simulink model "Simulation"  (R2016a)
settings: Solver=FixedStepAuto  StartTime=0.0  StopTime=20  FixedStep=0.01  RelTol=1e-3
undefined symbols (not defined in the file or in its folder): beta, g0, g1, g2, g3, gamma, kappa, landa, nu
(part 2 of 30)

== matlab function Simulation/Ueq ==
  data: e input; edot input; xddd input; despar input; landa input; S input; y1 output; theta input; thetadot input; y2 output; y3 output; y4 output; y5 output; y6 output
function [y1,y2,y3,y4,y5,y6] = fcn(e,edot,xddd,despar,landa,S,theta,thetadot)

y=zeros(6,1)
p1=despar(1)*((abs(e(1)))^despar(5))*sign(e(1))+despar(2)*e(1)+despar(3)*despar(6)*(abs(e(1)))^(despar(6)-1)*edot(1);
p2=despar(1)*((abs(e(2)))^despar(5))*sign(e(2))+despar(2)*e(2)+despar(3)*despar(6)*(abs(e(2)))^(despar(6)-1)*edot(2);
p3=despar(1)*((abs(e(3)))^despar(5))*sign(e(3))+despar(2)*e(3)+despar(3)*despar(6)*(abs(e(3)))^(despar(6)-1)*edot(3);
p4=despar(1)*((abs(e(4)))^despar(5))*sign(e(4))+despar(2)*e(4)+despar(3)*despar(6)*(abs(e(4)))^(despar(6)-1)*edot(4);
p5=despar(1)*((abs(e(5)))^despar(5))*sign(e(5))+despar(2)*e(5)+despar(3)*despar(6)*(abs(e(5)))^(despar(6)-1)*edot(5);
p6=despar(1)*((abs(e(6)))^despar(5))*sign(e(6))+despar(2)*e(6)+despar(3)*despar(6)*(abs(e(6)))^(despar(6)-1)*edot(6);

part=[p1 p2 p3 p4 p5 p6]';

theta1=theta(1)
theta2=theta(2)
theta3=theta(3)
theta4=theta(4)
theta5=theta(5)
theta6=theta(6)

thetadot1=thetadot(1)
thetadot2=thetadot(2)
thetadot3=thetadot(3)
thetadot4=thetadot(4)
thetadot5=thetadot(5)
thetadot6=thetadot(6)

MM=[ 0.1*cos(theta2 + theta3)^2 + (0.1*cos(theta2)*cos(theta3)*cos(theta6)*sin(theta4) - 0.1*cos(theta6)*sin(theta2)*sin(theta3)*sin(theta4) + 0.1*cos(theta2)*sin(theta3)*sin(theta5)*sin(theta6) + 0.1*cos(theta3)*sin(theta2)*sin(theta5)*sin(theta6) - 0.1*cos(theta2)*cos(theta3)*cos(theta4)*cos(theta5)*sin(theta6) + 0.1*cos(theta4)*cos(theta5)*sin(theta2)*sin(theta3)*sin(theta6))*(cos(theta2)*cos(theta3)*cos(theta6)*sin(theta4) - 1.0*cos(theta6)*sin(theta2)*sin(theta3)*sin(theta4) + cos(theta2)*sin(theta3)*sin(theta5)*sin(theta6) + cos(theta3)*sin(theta2)*sin(theta5)*sin(theta6) - 1.0*cos(theta2)*cos(theta3)*cos(theta4)*cos(theta5)*sin(theta6) + cos(theta4)*cos(theta5)*sin(theta2)*sin(theta3)*sin(theta6)) + 0.2*sin(theta2 + theta3)^2 + (0.2*cos(theta2)*sin(theta4)*sin(theta5) + 0.4*sin(theta2)*sin(theta3)*sin(theta4) - 0.4*cos(theta2)*cos(theta3)*sin(theta4) + 0.4*cos(theta2)*cos(theta3)*cos(theta6)*sin(theta4) + 0.4*cos(theta2)*cos(theta3)*sin(theta4)*sin(theta5) - 0.4*cos(theta6)*sin(theta2)*sin(theta3)*sin(theta4) + 0.4*cos(theta2)*sin(theta3)*sin(theta5)*sin(theta6) + 0.4*cos(theta3)*sin(theta2)*sin(theta5)*sin(theta6) - 0.4*sin(theta2)*sin(theta3)*sin(theta4)*sin(theta5) - 0.4*cos(theta2)*cos(theta3)*cos(theta4)*cos(theta5)*sin(theta6) + 0.4*cos(theta4)*cos(theta5)*sin(theta2)*sin(theta3)*sin(theta6))^2 + 0.14*cos(theta2)^2 + 0.1*sin(theta2)^2 + (cos(theta2)*sin(theta3)*sin(theta5) + cos(theta3)*sin(theta2)*sin(theta5) - 1.0*cos(theta2)*cos(theta3)*cos(theta4)*cos(theta5) + cos(theta4)*cos(theta5)*sin(theta2)*sin(theta3))*(0.1*cos(theta2)*sin(theta3)*sin(theta5) + 0.1*cos(theta3)*sin(theta2)*sin(theta5) - 0.1*cos(theta2)*cos(theta3)*cos(theta4)*cos(theta5) + 0.1*cos(theta4)*cos(theta5)*sin(theta2)*sin(theta3)) + 2.0*(cos(theta2)*cos(theta5)*sin(theta3) + cos(theta3)*cos(theta5)*sin(theta2) + cos(theta2)*cos(theta3)*cos(theta4)*sin(theta5) - 1.0*cos(theta4)*sin(theta2)*sin(theta3)*sin(theta5))*(0.1*cos(theta2)*cos(theta5)*sin(theta3) + 0.1*cos(theta3)*cos(theta5)*sin(theta2) + 0.1*cos(theta2)*cos(theta3)*cos(theta4)*sin(theta5) - 0.1*cos(theta4)*sin(theta2)*sin(theta3)*sin(theta5)) + 0.04*cos(theta4)^2*(2.0*cos(theta2 + theta3) + cos(theta2))^2 + 0.1*cos(theta2 + theta3)^2*cos(theta4)^2 + 0.2*cos(theta2 + theta3)^2*sin(theta4)^2 + (0.1*cos(theta2)*cos(theta6)*sin(theta3)*sin(theta5) - 0.1*cos(theta2)*cos(theta3)*sin(theta4)*sin(theta6) + 0.1*cos(theta3)*cos(theta6)*sin(theta2)*sin(theta5) + 0.1*sin(theta2)*sin(theta3)*sin(theta4)*sin(theta6) - 0.1*cos(theta2)*cos(theta3)*cos(theta4)*cos(theta5)*cos(theta6) + 0.1*cos(theta4)*cos(theta5)*cos(theta6)*sin(theta2)*sin(theta3))*(cos(theta2)*cos(theta6)*sin(theta3)*sin(theta5) - 1.0*cos(theta2)*cos(theta3)*sin(theta4)*sin(theta6) + cos(theta3)*cos(theta6)*sin(theta2)*sin(theta5) + sin(theta2)*sin(theta3)*sin(theta4)*sin(theta6) - 1.0*cos(theta2)*cos(theta3)*cos(theta4)*cos(theta5)*cos(theta6) + cos(theta4)*cos(theta5)*cos(theta6)*sin(theta2)*sin(theta3)) + 0.04*cos(theta4)^2*(cos(theta2 + theta3) + cos(theta2))^2 + 0.04*sin(theta4)^2*(cos(theta2 + theta3) + cos(theta2))^2 + (0.2*cos(theta2)*cos(theta5)*cos(theta6)*sin(theta4) - 0.4*cos(theta2)*cos(theta3)*cos(theta4)*sin(theta6) - 0.2*cos(theta2)*cos(theta4)*sin(theta6) + 0.4*cos(theta2)*cos(theta5)*sin(theta3)*sin(theta6) + 0.4*cos(theta3)*cos(theta5)*sin(theta2)*sin(theta6) + 0.4*cos(theta4)*sin(theta2)*sin(theta3)*sin(theta6) + 0.4*cos(theta2)*cos(theta3)*cos(theta5)*cos(theta6)*sin(theta4) + 0.4*cos(theta2)*cos(theta3)*cos(theta4)*sin(theta5)*sin(theta6) - 0.4*cos(theta5)*cos(theta6)*sin(theta2)*sin(theta3)*sin(theta4) - 0.4*cos(theta4)*sin(theta2)*sin(theta3)*sin(theta5)*sin(theta6))^2 + (0.2*cos(theta2)*cos(theta4)*cos(theta6) + 0.4*cos(theta2)*cos(theta5)*sin(theta3) + 0.4*cos(theta3)*cos(theta5)*sin(theta2) + 0.4*cos(theta2)*cos(theta3)*cos(theta4)*cos(theta6) + 0.4*cos(theta2)*cos(theta3)*cos(theta4)*sin(theta5) - 0.4*cos(theta2)*cos(theta5)*cos(theta6)*sin(theta3) - 0.4*cos(theta3)*cos(theta5)*cos(theta6)*sin(theta2) - 0.4*cos(theta4)*cos(theta6)*sin(theta2)*sin(theta3) + 0.2*cos(theta2)*cos(theta5)*sin(theta4)*sin(theta6) - 0.4*cos(theta4)*sin(theta2)*sin(theta3)*sin(theta5) - 0.4*cos(theta2)*cos(theta3)*cos(theta4)*cos(theta6)*sin(theta5) + 0.4*cos(theta2)*cos(theta3)*cos(theta5)*sin(theta4)*sin(theta6) + 0.4*cos(theta4)*cos(theta6)*sin(theta2)*sin(theta3)*sin(theta5) - 0.4*cos(theta5)*sin(theta2)*sin(theta3)*sin(theta4)*sin(theta6))^2 + 0.04*cos(theta5)^2*sin(theta4)^2*(2.0*cos(theta2 + theta3) + cos(theta2))^2 + 0.04*sin(theta4)^2*sin(theta5)^2*(2.0*cos(theta2 + theta3) + cos(theta2))^2 + 0.1, 0.16*cos(theta2)*cos(theta3)*cos(theta4)*sin(theta4) - 0.08*cos(theta4)*sin(theta2)*sin(theta6) - 0.08*cos(theta5)*sin(theta2)*sin(theta4) + 0.16*cos(theta2)*cos(theta3)*cos(theta5)*sin(theta6) - 0.16*cos(theta2)*cos(theta5)*sin(theta3)*sin(theta4) - 0.16*cos(theta3)*cos(theta5)*sin(theta2)*sin(theta4) - 0.16*cos(theta2)*cos(theta4)*sin(theta3)*sin(theta6) - 0.16*cos(theta3)*cos(theta4)*sin(theta2)*sin(theta6) + 0.08*cos(theta5)*cos(theta6)*sin(theta2)*sin(theta4) - 0.16*cos(theta4)*sin(theta2)*sin(theta3)*sin(theta4) - 0.16*cos(theta5)*sin(theta2)*sin(theta3)*sin(theta6) - 0.16*cos(theta2)*cos(theta3)*cos(theta4)*cos(theta5)^2*sin(theta4) - 0.16*cos(theta2)*cos(theta3)*cos(theta4)*cos(theta6)^2*sin(theta4) - 0.32*cos(theta2)*cos(theta3)*cos(theta4)^2*cos(theta5)*sin(theta6) + 0.16*cos(theta4)*cos(theta5)^2*sin(theta2)*sin(theta3)*sin(theta4) + 0.16*cos(theta4)*cos(theta6)^2*sin(theta2)*sin(theta3)*sin(theta4) + 0.32*cos(theta4)^2*cos(theta5)*sin(theta2)*sin(theta3)*sin(theta6) - 0.16*cos(theta2)*cos(theta3)*cos(theta5)*cos(theta6)*sin(theta6) + 0.16*cos(theta2)*cos(theta5)*cos(theta6)*sin(theta3)*sin(theta4) + 0.16*cos(theta3)*cos(theta5)*cos(theta6)*sin(theta2)*sin(theta4) + 0.16*cos(theta2)*cos(theta5)*sin(theta3)*sin(theta4)*sin(theta5) + 0.16*cos(theta3)*cos(theta5)*sin(theta2)*sin(theta4)*sin(theta5) + 0.16*cos(theta2)*cos(theta4)*sin(theta3)*sin(theta5)*sin(theta6) + 0.16*cos(theta3)*cos(theta4)*sin(theta2)*sin(theta5)*sin(theta6) + 0.16*cos(theta5)*cos(theta6)*sin(theta2)*sin(theta3)*sin(theta6) - 0.16*cos(theta2)*cos(theta3)*cos(theta4)*cos(theta5)^2*cos(theta6)^2*sin(theta4) + 0.16*cos(theta4)*cos(theta5)^2*cos(theta6)^2*sin(theta2)*sin(theta3)*sin(theta4) - 0.32*cos(theta2)*cos(theta5)*cos(theta6)*sin(theta3)*sin(theta4)*sin(theta5) - 0.32*cos(theta3)*cos(theta5)*cos(theta6)*sin(theta2)*sin(theta4)*sin(theta5) - 0.16*cos(theta2)*cos(theta4)*cos(theta6)*sin(theta3)*sin(theta5)*sin(theta6) - 0.16*cos(theta3)*cos(theta4)*cos(theta6)*sin(theta2)*sin(theta5)*sin(theta6) + 0.32*cos(theta2)*cos(theta3)*cos(theta4)*cos(theta5)^2*cos(theta6)*sin(theta4) + 0.32*cos(theta2)*cos(theta3)*cos(theta4)^2*cos(theta5)*cos(theta6)*sin(theta6) - 0.32*cos(theta4)*cos(theta5)^2*cos(theta6)*sin(theta2)*sin(theta3)*sin(theta4) + 0.16*cos(theta2)*cos(theta5)*cos(theta6)^2*sin(theta3)*sin(theta4)*sin(theta5) + 0.16*cos(theta3)*cos(theta5)*cos(theta6)^2*sin(theta2)*sin(theta4)*sin(theta5) - 0.32*cos(theta4)^2*cos(theta5)*cos(theta6)*sin(theta2)*sin(theta3)*sin(theta6), 0.16*cos(theta2)*cos(theta3)*cos(theta4)*sin(theta4) + 0.16*cos(theta2)*cos(theta3)*cos(theta5)*sin(theta6) - 0.16*cos(theta2)*cos(theta5)*sin(theta3)*sin(theta4) - 0.16*cos(theta3)*cos(theta5)*sin(theta2)*sin(theta4) - 0.16*cos(theta2)*cos(theta4)*sin(theta3)*sin(theta6) - 0.16*cos(theta3)*cos(theta4)*sin(theta2)*sin(theta6) - 0.16*cos(theta4)*sin(theta2)*sin(theta3)*sin(theta4) - 0.16*cos(theta5)*sin(theta2)*sin(theta3)*sin(theta6) - 0.16*cos(theta2)*cos(theta3)*cos(theta4)*cos(theta5)^2*sin(theta4) - 0.16*cos(theta2)*cos(theta3)*cos(theta4)*cos(theta6)^2*sin(theta4) - 0.32*cos(theta2)*cos(theta3)*cos(theta4)^2*cos(theta5)*sin(theta6) + 0.16*cos(theta4)*cos(theta5)^2*sin(theta2)*sin(theta3)*sin(theta4) + 0.16*cos(theta4)*cos(theta6)^2*sin(theta2)*sin(theta3)*sin(theta4) + 0.32*cos(theta4)^2*cos(theta5)*sin(theta2)*sin(theta3)*sin(theta6) - 0.16*cos(theta2)*cos(theta3)*cos(theta5)*cos(theta6)*sin(theta6) + 0.16*cos(theta2)*cos(theta5)*cos(theta6)*sin(theta3)*sin(theta4) + 0.16*cos(theta3)*cos(theta5)*cos(theta6)*sin(theta2)*sin(theta4) + 0.16*cos(theta2)*cos(theta5)*sin(theta3)*sin(theta4)*sin(theta5) + 0.16*cos(theta3)*cos(theta5)*sin(theta2)*sin(theta4)*sin(theta5) + 0.16*cos(theta2)*cos(theta4)*sin(theta3)*sin(theta5)*sin(theta6) + 0.16*cos(theta3)*cos(theta4)*sin(theta2)*sin(theta5)*sin(theta6) + 0.16*cos(theta5)*cos(theta6)*sin(theta2)*sin(theta3)*sin(theta6) - 0.16*cos(theta2)*cos(theta3)*cos(theta4)*cos(theta5)^2*cos(theta6)^2*sin(theta4) + 0.16*cos(theta4)*cos(theta5)^2*cos(theta6)^2*sin(theta2)*sin(theta3)*sin(theta4) - 0.32*cos(theta2)*cos(theta5)*cos(theta6)*sin(theta3)*sin(theta4)*sin(theta5) - 0.32*cos(theta3)*cos(theta5)*cos(theta6)*sin(theta2)*sin(theta4)*sin(theta5) - 0.16*cos(theta2)*cos(theta4)*cos(theta6)*sin(theta3)*sin(theta5)*sin(theta6) - 0.16*cos(theta3)*cos(theta4)*cos(theta6)*sin(theta2)*sin(theta5)*sin(theta6) + 0.32*cos(theta2)*cos(theta3)*cos(theta4)*cos(theta5)^2*cos(theta6)*sin(theta4) + 0.32*cos(theta2)*cos(theta3)*cos(theta4)^2*cos(theta5)*cos(theta6)*sin(theta6) - 0.32*cos(theta4)*cos(theta5)^2*cos(theta6)*sin(theta2)*sin(theta3)*sin(theta4) + 0.16*cos(theta2)*cos(theta5)*cos(theta6)^2*sin(theta3)*sin(theta4)*sin(theta5) + 0.16*cos(theta3)*cos(theta5)*cos(theta6)^2*sin(theta2)*sin(theta4)*sin(theta5) - 0.32*cos(theta4)^2*cos(theta5)*cos(theta6)*sin(theta2)*sin(theta3)*sin(theta6), 0.46*cos(theta2)*sin(theta3) + 0.46*cos(theta3)*sin(theta2) + 0.08*cos(theta2)*sin(theta4)*sin(theta6) + 0.16*cos(theta2)*cos(theta5)^2*sin(theta3) + 0.16*cos(theta3)*cos(theta5)^2*sin(theta2) - 0.16*cos(theta2)*cos(theta6)^2*sin(theta3) - 0.16*cos(theta3)*cos(theta6)^2*sin(theta2) - 0.08*cos(theta2)*cos(theta4)*cos(theta5) - 0.32*cos(theta2)*cos(theta5)^2*cos(theta6)*sin(theta3) - 0.32*cos(theta3)*cos(theta5)^2*cos(theta6)*sin(theta2) + 0.16*cos(theta2)*cos(theta5)^2*cos(theta6)^2*sin(theta3) + 0.16*cos(theta3)*cos(theta5)^2*cos(theta6)^2*sin(theta2) - 0.16*cos(theta2)*cos(theta3)*cos(theta4)*cos(theta5) + 0.08*cos(theta2)*cos(theta4)*cos(theta5)*cos(theta6) + 0.16*cos(theta4)*cos(theta5)*sin(theta2)*sin(theta3) + 0.16*cos(theta2)*cos(theta3)*sin(theta4)*sin(theta6) - 0.16*sin(theta2)*sin(theta3)*sin(theta4)*sin(theta6) + 0.16*cos(theta2)*cos(theta3)*cos(theta4)*cos(theta5)*cos(theta6) + 0.16*cos(theta2)*cos(theta3)*cos(theta4)*cos(theta5)*sin(theta5) - 0.16*cos(theta4)*cos(theta5)*cos(theta6)*sin(theta2)*sin(theta3) - 0.16*cos(theta4)*cos(theta5)*sin(theta2)*sin(theta3)*sin(theta5) - 0.16*cos(theta2)*cos(theta3)*sin(theta4)*sin(theta5)*sin(theta6) + 0.16*sin(theta2)*sin(theta3)*sin(theta4)*sin(theta5)*sin(theta6) - 0.32*cos(theta2)*cos(theta3)*cos(theta4)*cos(theta5)*cos(theta6)*sin(theta5) + 0.32*cos(theta4)*cos(theta5)*cos(theta6)*sin(theta2)*sin(theta3)*sin(theta5) + 0.16*cos(theta2)*cos(theta3)*cos(theta6)*sin(theta4)*sin(theta5)*sin(theta6) - 0.16*cos(theta6)*sin(theta2)*sin(theta3)*sin(theta4)*sin(theta5)*sin(theta6) + 0.16*cos(theta2)*cos(theta3)*cos(theta4)*cos(theta5)*cos(theta6)^2*sin(theta5) - 0.16*cos(theta4)*cos(theta5)*cos(theta6)^2*sin(theta2)*sin(theta3)*sin(theta5), 0.08*cos(theta2)*sin(theta4)*sin(theta5) + 0.36*sin(theta2)*sin(theta3)*sin(theta4) - 0.36*cos(theta2)*cos(theta3)*sin(theta4) - 0.16*cos(theta2)*cos(theta3)*cos(theta6)^2*sin(theta4) + 0.16*cos(theta6)^2*sin(theta2)*sin(theta3)*sin(theta4) + 0.32*cos(theta2)*cos(theta3)*cos(theta6)*sin(theta4) + 0.16*cos(theta2)*cos(theta3)*sin(theta4)*sin(theta5) - 0.08*cos(theta2)*cos(theta6)*sin(theta4)*sin(theta5) - 0.32*cos(theta6)*sin(theta2)*sin(theta3)*sin(theta4) + 0.16*cos(theta2)*sin(theta3)*sin(theta5)*sin(theta6) + 0.16*cos(theta3)*sin(theta2)*sin(theta5)*sin(theta6) - 0.16*sin(theta2)*sin(theta3)*sin(theta4)*sin(theta5) - 0.16*cos(theta2)*cos(theta3)*cos(theta4)*cos(theta5)*sin(theta6) - 0.16*cos(theta2)*cos(theta3)*cos(theta6)*sin(theta4)*sin(theta5) + 0.16*cos(theta4)*cos(theta5)*sin(theta2)*sin(theta3)*sin(theta6) - 0.16*cos(theta2)*cos(theta6)*sin(theta3)*sin(theta5)*sin(theta6) - 0.16*cos(theta3)*cos(theta6)*sin(theta2)*sin(theta5)*sin(theta6) + 0.16*cos(theta6)*sin(theta2)*sin(theta3)*sin(theta4)*sin(theta5) + 0.16*cos(theta2)*cos(theta3)*cos(theta4)*cos(theta5)*cos(theta6)*sin(theta6) - 0.16*cos(theta4)*cos(theta5)*cos(theta6)*sin(theta2)*sin(theta3)*sin(theta6), 0.08*cos(theta2)*cos(theta4)*cos(theta6) + 0.26*cos(theta2)*cos(theta5)*sin(theta3) + 0.26*cos(theta3)*cos(theta5)*sin(theta2) + 0.16*cos(theta2)*cos(theta3)*cos(theta4)*cos(theta6) + 0.26*cos(theta2)*cos(theta3)*cos(theta4)*sin(theta5) - 0.16*cos(theta2)*cos(theta5)*cos(theta6)*sin(theta3) - 0.16*cos(theta3)*cos(theta5)*cos(theta6)*sin(theta2) - 0.16*cos(theta4)*cos(theta6)*sin(theta2)*sin(theta3) + 0.08*cos(theta2)*cos(theta5)*sin(theta4)*sin(theta6) - 0.26*cos(theta4)*sin(theta2)*sin(theta3)*sin(theta5) - 0.16*cos(theta2)*cos(theta3)*cos(theta4)*cos(theta6)*sin(theta5) + 0.16*cos(theta2)*cos(theta3)*cos(theta5)*sin(theta4)*sin(theta6) + 0.16*cos(theta4)*cos(theta6)*sin(theta2)*sin(theta3)*sin(theta5) - 0.16*cos(theta5)*sin(theta2)*sin(theta3)*sin(theta4)*sin(theta6);
                                                                                                                                                                                                                                                                                                                                                                                                                                                                                                                                                                                                                                                                                                                                                                                                                                                                                                                                                                                                                                                                                                                                                                                                                                                                                                                                                                                                                                                                                                                                                                                                                                                                                                                                                                                                                                                                                                                                                                                                                                                                                                                                                                       0.16*cos(theta2)*cos(theta3)*cos(theta4)*sin(theta4) - 0.08*cos(theta4)*sin(theta2)*sin(theta6) - 0.08*cos(theta5)*sin(theta2)*sin(theta4) + 0.16*cos(theta2)*cos(theta3)*cos(theta5)*sin(theta6) - 0.16*cos(theta2)*cos(theta5)*sin(theta3)*sin(theta4) - 0.16*cos(theta3)*cos(theta5)*sin(theta2)*sin(theta4) - 0.16*cos(theta2)*cos(theta4)*sin(theta3)*sin(theta6) - 0.16*cos(theta3)*cos(theta4)*sin(theta2)*sin(theta6) + 0.08*cos(theta5)*cos(theta6)*sin(theta2)*sin(theta4) - 0.16*cos(theta4)*sin(theta2)*sin(theta3)*sin(theta4) - 0.16*cos(theta5)*sin(theta2)*sin(theta3)*sin(theta6) - 0.16*cos(theta2)*cos(theta3)*cos(theta4)*cos(theta5)^2*sin(theta4) - 0.16*cos(theta2)*cos(theta3)*cos(theta4)*cos(theta6)^2*sin(theta4) - 0.32*cos(theta2)*cos(theta3)*cos(theta4)^2*cos(theta5)*sin(theta6) + 0.16*cos(theta4)*cos(theta5)^2*sin(theta2)*sin(theta3)*sin(theta4) + 0.16*cos(theta4)*cos(theta6)^2*sin(theta2)*sin(theta3)*sin(theta4) + 0.32*cos(theta4)^2*cos(theta5)*sin(theta2)*sin(theta3)*sin(theta6) - 0.16*cos(theta2)*cos(theta3)*cos(theta5)*cos(theta6)*sin(theta6) + 0.16*cos(theta2)*cos(theta5)*cos(theta6)*sin(theta3)*sin(theta4) + 0.16*cos(theta3)*cos(theta5)*cos(theta6)*sin(theta2)*sin(theta4) + 0.16*cos(theta2)*cos(theta5)*sin(theta3)*sin(theta4)*sin(theta5) + 0.16*cos(theta3)*cos(theta5)*sin(theta2)*sin(theta4)*sin(theta5) + 0.16*cos(theta2)*cos(theta4)*sin(theta3)*sin(theta5)*sin(theta6) + 0.16*cos(theta3)*cos(theta4)*sin(theta2)*sin(theta5)*sin(theta6) + 0.16*cos(theta5)*cos(theta6)*sin(theta2)*sin(theta3)*sin(theta6) - 0.16*cos(theta2)*cos(theta3)*cos(theta4)*cos(theta5)^2*cos(theta6)^2*sin(theta4) + 0.16*cos(theta4)*cos(theta5)^2*cos(theta6)^2*sin(theta2)*sin(theta3)*sin(theta4) - 0.32*cos(theta2)*cos(theta5)*cos(theta6)*sin(theta3)*sin(theta4)*sin(theta5) - 0.32*cos(theta3)*cos(theta5)*cos(theta6)*sin(theta2)*sin(theta4)*sin(theta5) - 0.16*cos(theta2)*cos(theta4)*cos(theta6)*sin(theta3)*sin(theta5)*sin(theta6) - 0.16*cos(theta3)*cos(theta4)*cos(theta6)*sin(theta2)*sin(theta5)*sin(theta6) + 0.32*cos(theta2)*cos(theta3)*cos(theta4)*cos(theta5)^2*cos(theta6)*sin(theta4) + 0.32*cos(theta2)*cos(theta3)*cos(theta4)^2*cos(theta5)*cos(theta6)*sin(theta6) - 0.32*cos(theta4)*cos(theta5)^2*cos(theta6)*sin(theta2)*sin(theta3)*sin(theta4) + 0.16*cos(theta2)*cos(theta5)*cos(theta6)^2*sin(theta3)*sin(theta4)*sin(theta5) + 0.16*cos(theta3)*cos(theta5)*cos(theta6)^2*sin(theta2)*sin(theta4)*sin(theta5) - 0.32*cos(theta4)^2*cos(theta5)*cos(theta6)*sin(theta2)*sin(theta3)*sin(theta6),                                                                                                                                                                                                                                                                                                                                                                                                                                                                                                                                                                                                                                                                                                                                                                                                                                                                                                                                                                                                                         (0.1*cos(theta4)*cos(theta6) + 0.1*cos(theta5)*sin(theta4)*sin(theta6))*(cos(theta4)*cos(theta6) + cos(theta5)*sin(theta4)*sin(theta6)) + (0.4*cos(theta4)*cos(theta5) - 0.2*sin(theta3)*sin(theta5) + 0.2*cos(theta3)*cos(theta4)*cos(theta5))^2 + (0.4*sin(theta4)*sin(theta6) + 0.2*cos(theta3)*sin(theta4)*sin(theta6) - 0.2*cos(theta6)*sin(theta3)*sin(theta5) - 0.4*sin(theta4)*sin(theta5)*sin(theta6) + 0.4*cos(theta4)*cos(theta5)*cos(theta6) + 0.2*cos(theta3)*cos(theta4)*cos(theta5)*cos(theta6))^2 + (0.2*cos(theta5)*sin(theta3) + 0.4*cos(theta4)*sin(theta5) + 0.2*cos(theta3)*cos(theta4)*sin(theta5))^2 + 0.04*cos(theta3)^2 + 0.2*cos(theta4)^2 + 0.08*sin(theta3)^2 + 0.1*sin(theta4)^2 + (0.1*cos(theta4)*sin(theta6) - 0.1*cos(theta5)*cos(theta6)*sin(theta4))*(cos(theta4)*sin(theta6) - 1.0*cos(theta5)*cos(theta6)*sin(theta4)) + 0.04*cos(theta4)^2*(cos(theta3) + 1.0)^2 + 0.04*sin(theta4)^2*(cos(theta3) + 1.0)^2 + 0.04*sin(theta4)^2*(cos(theta3) + 2.0)^2 + (0.4*cos(theta4)*cos(theta6) - 0.4*cos(theta4) + 0.2*cos(theta5)*sin(theta3) + 0.4*cos(theta4)*sin(theta5) + 0.4*cos(theta5)*sin(theta4)*sin(theta6) + 0.2*cos(theta3)*cos(theta4)*sin(theta5))^2 + (0.4*cos(theta6)*sin(theta4) + 0.4*sin(theta4)*sin(theta5) - 0.4*cos(theta6)*sin(theta4)*sin(theta5) + 0.2*sin(theta3)*sin(theta5)*sin(theta6) + 0.2*cos(theta3)*cos(theta6)*sin(theta4) - 0.4*cos(theta4)*cos(theta5)*sin(theta6) - 0.2*cos(theta3)*cos(theta4)*cos(theta5)*sin(theta6))^2 + 0.1*cos(theta5)^2*sin(theta4)^2 + 0.2*sin(theta4)^2*sin(theta5)^2 + 0.2,                                                                                                                                                                                                                                                                                                                                                                                                                                                                                                                                                                                                                                                                                                                                                                                                                                                                                                                                                                                                                                                                                                                                                                                                                                                                                                                                                                                                                                                                                                                                                                                                                                                                                                                    0.2*cos(theta3) - 0.32*cos(theta6) - 0.32*sin(theta5) - 0.08*cos(theta3)*sin(theta5) + 0.32*cos(theta6)*sin(theta5) - 0.16*cos(theta4)^2 - 0.16*cos(theta5)^2 + 0.32*cos(theta5)^2*cos(theta6) + 0.16*cos(theta4)^2*cos(theta5)^2 + 0.16*cos(theta4)^2*cos(theta6)^2 - 0.16*cos(theta5)^2*cos(theta6)^2 + 0.16*cos(theta4)^2*cos(theta5)^2*cos(theta6)^2 + 0.08*sin(theta3)*sin(theta4)*sin(theta6) - 0.32*cos(theta4)^2*cos(theta5)^2*cos(theta6) - 0.08*cos(theta4)*cos(theta5)*sin(theta3) + 0.08*cos(theta3)*cos(theta6)*sin(theta5) + 0.08*cos(theta4)*cos(theta5)*cos(theta6)*sin(theta3) - 0.32*cos(theta4)*cos(theta5)*sin(theta4)*sin(theta6) + 0.32*cos(theta4)*cos(theta5)*cos(theta6)*sin(theta4)*sin(theta6) + 1.08,                                                                                                                                                                                                                                                                                                                                                                                                                                                                                                                                                                                                                                                                                                                                                                                                                                                                                                                                                                                                                                                                                                                                                                                                                                                                                                                                                                                                                                                                                                                                                                                                        -(2*(cos(theta5)*sin(theta4) + cos(theta4)*sin(theta6) - 1.0*cos(theta5)*cos(theta6)*sin(theta4))*(cos(theta3) - 2.0*sin(theta5) + 2.0*cos(theta6)*sin(theta5) + 2.0))/25,                                                                                                                                                                                                                                                                                                                                                                                                                                                                                                                                                                                                                                                                                                                                                                                                             0.1*cos(theta4) + (0.4*cos(theta6) - 0.4)*(0.4*cos(theta4)*cos(theta6) - 0.4*cos(theta4) + 0.2*cos(theta5)*sin(theta3) + 0.4*cos(theta4)*sin(theta5) + 0.4*cos(theta5)*sin(theta4)*sin(theta6) + 0.2*cos(theta3)*cos(theta4)*sin(theta5)) + cos(theta6)*(0.1*cos(theta4)*cos(theta6) + 0.1*cos(theta5)*sin(theta4)*sin(theta6)) + sin(theta6)*(0.1*cos(theta4)*sin(theta6) - 0.1*cos(theta5)*cos(theta6)*sin(theta4)),                                                                                                                                                                                                                                                                                                                                                                                                                                                                                                              0.16*cos(theta6)*sin(theta4) + 0.26*sin(theta4)*sin(theta5) - 0.16*cos(theta6)*sin(theta4)*sin(theta5) + 0.08*sin(theta3)*sin(theta5)*sin(theta6) + 0.08*cos(theta3)*cos(theta6)*sin(theta4) - 0.16*cos(theta4)*cos(theta5)*sin(theta6) - 0.08*cos(theta3)*cos(theta4)*cos(theta5)*sin(theta6);
                                                                                                                                                                                                                                                                                                                                                                                                                                                                                                                                                                                                                                                                                                                                                                                                                                                                                                                                                                                                                                                                                                                                                                                                                                                                                                                                                                                                                                                                                                                                                                                                                                                                                                                                                                                                                                                                                                                                                                                                                                                                                                                                                                                                                                                                                                                   0.16*cos(theta2)*cos(theta3)*cos(theta4)*sin(theta4) + 0.16*cos(theta2)*cos(theta3)*cos(theta5)*sin(theta6) - 0.16*cos(theta2)*cos(theta5)*sin(theta3)*sin(theta4) - 0.16*cos(theta3)*cos(theta5)*sin(theta2)*sin(theta4) - 0.16*cos(theta2)*cos(theta4)*sin(theta3)*sin(theta6) - 0.16*cos(theta3)*cos(theta4)*sin(theta2)*sin(theta6) - 0.16*cos(theta4)*sin(theta2)*sin(theta3)*sin(theta4) - 0.16*cos(theta5)*sin(theta2)*sin(theta3)*sin(theta6) - 0.16*cos(theta2)*cos(theta3)*cos(theta4)*cos(theta5)^2*sin(theta4) - 0.16*cos(theta2)*cos(theta3)*cos(theta4)*cos(theta6)^2*sin(theta4) - 0.32*cos(theta2)*cos(theta3)*cos(theta4)^2*cos(theta5)*sin(theta6) + 0.16*cos(theta4)*cos(theta5)^2*sin(theta2)*sin(theta3)*sin(theta4) + 0.16*cos(theta4)*cos(theta6)^2*sin(theta2)*sin(theta3)*sin(theta4) + 0.32*cos(theta4)^2*cos(theta5)*sin(theta2)*sin(theta3)*sin(theta6) - 0.16*cos(theta2)*cos(theta3)*cos(theta5)*cos(theta6)*sin(theta6) + 0.16*cos(theta2)*cos(theta5)*cos(theta6)*sin(theta3)*sin(theta4) + 0.16*cos(theta3)*cos(theta5)*cos(theta6)*sin(theta2)*sin(theta4) + 0.16*cos(theta2)*cos(theta5)*sin(theta3)*sin(theta4)*sin(theta5) + 0.16*cos(theta3)*cos(theta5)*sin(theta2)*sin(theta4)*sin(theta5) + 0.16*cos(theta2)*cos(theta4)*sin(theta3)*sin(theta5)*sin(theta6) + 0.16*cos(theta3)*cos(theta4)*sin(theta2)*sin(theta5)*sin(theta6) + 0.16*cos(theta5)*cos(theta6)*sin(theta2)*sin(theta3)*sin(theta6) - 0.16*cos(theta2)*cos(theta3)*cos(theta4)*cos(theta5)^2*cos(theta6)^2*sin(theta4) + 0.16*cos(theta4)*cos(theta5)^2*cos(theta6)^2*sin(theta2)*sin(theta3)*sin(theta4) - 0.32*cos(theta2)*cos(theta5)*cos(theta6)*sin(theta3)*sin(theta4)*sin(theta5) - 0.32*cos(theta3)*cos(theta5)*cos(theta6)*sin(theta2)*sin(theta4)*sin(theta5) - 0.16*cos(theta2)*cos(theta4)*cos(theta6)*sin(theta3)*sin(theta5)*sin(theta6) - 0.16*cos(theta3)*cos(theta4)*cos(theta6)*sin(theta2)*sin(theta5)*sin(theta6) + 0.32*cos(theta2)*cos(theta3)*cos(theta4)*cos(theta5)^2*cos(theta6)*sin(theta4) + 0.32*cos(theta2)*cos(theta3)*cos(theta4)^2*cos(theta5)*cos(theta6)*sin(theta6) - 0.32*cos(theta4)*cos(theta5)^2*cos(theta6)*sin(theta2)*sin(theta3)*sin(theta4) + 0.16*cos(theta2)*cos(theta5)*cos(theta6)^2*sin(theta3)*sin(theta4)*sin(theta5) + 0.16*cos(theta3)*cos(theta5)*cos(theta6)^2*sin(theta2)*sin(theta4)*sin(theta5) - 0.32*cos(theta4)^2*cos(theta5)*cos(theta6)*sin(theta2)*sin(theta3)*sin(theta6),                                                                                                                                                                                                                                                                                                                                                                                                                                                                                                                                                                                                                                                                                                                                                                                                                                                                                                                                                                                                                                                                                                                                                                                                                                                                                                                                                                                                                                                                                                                                                                                                                                                                                                                                                                                                                                                                 0.2*cos(theta3) - 0.32*cos(theta6) - 0.32*sin(theta5) - 0.08*cos(theta3)*sin(theta5) + 0.32*cos(theta6)*sin(theta5) - 0.16*cos(theta4)^2 - 0.16*cos(theta5)^2 + 0.32*cos(theta5)^2*cos(theta6) + 0.16*cos(theta4)^2*cos(theta5)^2 + 0.16*cos(theta4)^2*cos(theta6)^2 - 0.16*cos(theta5)^2*cos(theta6)^2 + 0.16*cos(theta4)^2*cos(theta5)^2*cos(theta6)^2 + 0.08*sin(theta3)*sin(theta4)*sin(theta6) - 0.32*cos(theta4)^2*cos(theta5)^2*cos(theta6) - 0.08*cos(theta4)*cos(theta5)*sin(theta3) + 0.08*cos(theta3)*cos(theta6)*sin(theta5) + 0.08*cos(theta4)*cos(theta5)*cos(theta6)*sin(theta3) - 0.32*cos(theta4)*cos(theta5)*sin(theta4)*sin(theta6) + 0.32*cos(theta4)*cos(theta5)*cos(theta6)*sin(theta4)*sin(theta6) + 1.08,                                                                                                                                                                                                                                                                                                                                                                                                                                                                                                                                                                                                                                                                                                                                                                                                                                                                                                                                                                                                                                                                                                                                                                                                                                                                                                                                                                                                                                                                                                                                                                (0.1*cos(theta4)*cos(theta6) + 0.1*cos(theta5)*sin(theta4)*sin(theta6))*(cos(theta4)*cos(theta6) + cos(theta5)*sin(theta4)*sin(theta6)) + (0.4*sin(theta4)*sin(theta6) - 0.4*sin(theta4)*sin(theta5)*sin(theta6) + 0.4*cos(theta4)*cos(theta5)*cos(theta6))^2 + 0.24*cos(theta4)^2 + 0.3*sin(theta4)^2 + (0.1*cos(theta4)*sin(theta6) - 0.1*cos(theta5)*cos(theta6)*sin(theta4))*(cos(theta4)*sin(theta6) - 1.0*cos(theta5)*cos(theta6)*sin(theta4)) + (0.4*cos(theta6)*sin(theta4) + 0.4*sin(theta4)*sin(theta5) - 0.4*cos(theta6)*sin(theta4)*sin(theta5) - 0.4*cos(theta4)*cos(theta5)*sin(theta6))^2 + (0.4*cos(theta4)*cos(theta6) - 0.4*cos(theta4) + 0.4*cos(theta4)*sin(theta5) + 0.4*cos(theta5)*sin(theta4)*sin(theta6))^2 + 0.16*cos(theta4)^2*cos(theta5)^2 + 0.16*cos(theta4)^2*sin(theta5)^2 + 0.1*cos(theta5)^2*sin(theta4)^2 + 0.2*sin(theta4)^2*sin(theta5)^2 + 0.1,                                                                                                                                                                                                                                                                                                                                                                                                                                                                                                                                                                                                                                                                                                                                                                                                                                                                                                                                                                                                                                                                                                                                                                                                                                                                                                                                                                                                                                                                                                                                                                                                                          -(4*(cos(theta6)*sin(theta5) - 1.0*sin(theta5) + 1.0)*(cos(theta5)*sin(theta4) + cos(theta4)*sin(theta6) - 1.0*cos(theta5)*cos(theta6)*sin(theta4)))/25,                                                                                                                                                                                                                                                                                                                                                                                                                                                                                                                                                                                                                                                                                                                                                                                                                                                                                                                                                                      0.36*cos(theta4) - 0.32*cos(theta4)*cos(theta6) - 0.16*cos(theta4)*sin(theta5) + 0.16*cos(theta4)*cos(theta6)^2 - 0.16*cos(theta5)*sin(theta4)*sin(theta6) + 0.16*cos(theta4)*cos(theta6)*sin(theta5) + 0.16*cos(theta5)*cos(theta6)*sin(theta4)*sin(theta6),                                                                                                                                                                                                                                                                                                                                                                                                                                                                                                                                                                                                                                                           0.16*cos(theta6)*sin(theta4) + 0.26*sin(theta4)*sin(theta5) - 0.16*cos(theta6)*sin(theta4)*sin(theta5) - 0.16*cos(theta4)*cos(theta5)*sin(theta6);
                                                                                                                                                                                                                                                                                                                                                                                                                                                                                                                                                                                                                                                                                                                                                                                                                                                                                                                                                                                                                                                                                                                                                                                                                                                                                                                                                                                                                                                                                                                                                                                                                                                                                                                                                                                                                                                                                                                                                                                                                                                                                                                                                                                                                                                                                                                                                                                                                                                                                                                                                                                                                                                                                                                                                                                                                                                                                                                                                                                       0.46*cos(theta2)*sin(theta3) + 0.46*cos(theta3)*sin(theta2) + 0.08*cos(theta2)*sin(theta4)*sin(theta6) + 0.16*cos(theta2)*cos(theta5)^2*sin(theta3) + 0.16*cos(theta3)*cos(theta5)^2*sin(theta2) - 0.16*cos(theta2)*cos(theta6)^2*sin(theta3) - 0.16*cos(theta3)*cos(theta6)^2*sin(theta2) - 0.08*cos(theta2)*cos(theta4)*cos(theta5) - 0.32*cos(theta2)*cos(theta5)^2*cos(theta6)*sin(theta3) - 0.32*cos(theta3)*cos(theta5)^2*cos(theta6)*sin(theta2) + 0.16*cos(theta2)*cos(theta5)^2*cos(theta6)^2*sin(theta3) + 0.16*cos(theta3)*cos(theta5)^2*cos(theta6)^2*sin(theta2) - 0.16*cos(theta2)*cos(theta3)*cos(theta4)*cos(theta5) + 0.08*cos(theta2)*cos(theta4)*cos(theta5)*cos(theta6) + 0.16*cos(theta4)*cos(theta5)*sin(theta2)*sin(theta3) + 0.16*cos(theta2)*cos(theta3)*sin(theta4)*sin(theta6) - 0.16*sin(theta2)*sin(theta3)*sin(theta4)*sin(theta6) + 0.16*cos(theta2)*cos(theta3)*cos(theta4)*cos(theta5)*cos(theta6) + 0.16*cos(theta2)*cos(theta3)*cos(theta4)*cos(theta5)*sin(theta5) - 0.16*cos(theta4)*cos(theta5)*cos(theta6)*sin(theta2)*sin(theta3) - 0.16*cos(theta4)*cos(theta5)*sin(theta2)*sin(theta3)*sin(theta5) - 0.16*cos(theta2)*cos(theta3)*sin(theta4)*sin(theta5)*sin(theta6) + 0.16*sin(theta2)*sin(theta3)*sin(theta4)*sin(theta5)*sin(theta6) - 0.32*cos(theta2)*cos(theta3)*cos(theta4)*cos(theta5)*cos(theta6)*sin(theta5) + 0.32*cos(theta4)*cos(theta5)*cos(theta6)*sin(theta2)*sin(theta3)*sin(theta5) + 0.16*cos(theta2)*cos(theta3)*cos(theta6)*sin(theta4)*sin(theta5)*sin(theta6) - 0.16*cos(theta6)*sin(theta2)*sin(theta3)*sin(theta4)*sin(theta5)*sin(theta6) + 0.16*cos(theta2)*cos(theta3)*cos(theta4)*cos(theta5)*cos(theta6)^2*sin(theta5) - 0.16*cos(theta4)*cos(theta5)*cos(theta6)^2*sin(theta2)*sin(theta3)*sin(theta5),                                                                                                                                                                                                                                                                                                                                                                                                                                                                                                                                                                                                                                                                                                                                                                                                                                                                                                                                                                                                                                                                                                                                                                                                                                                                                                                                                                                                                                                                                                                                                                                                                                                                                                                                                                                                                                                                                                                                                                                                                                                                                                                                                                                                                                                                                                                                                                                                                        -(2*(cos(theta5)*sin(theta4) + cos(theta4)*sin(theta6) - 1.0*cos(theta5)*cos(theta6)*sin(theta4))*(cos(theta3) - 2.0*sin(theta5) + 2.0*cos(theta6)*sin(theta5) + 2.0))/25,                                                                                                                                                                                                                                                                                                                                                                                                                                                                                                                                                                                                                                                                                                                                                                                                                                                                                                                                                                                                                                                                                                                                                                                                                                                                                                                                                                                                                                                                                                                                                                                                                                                                                                                                                                                                                                                                                                                                                                                                                                                                                                                                                                                                                                                                                             -(4*(cos(theta6)*sin(theta5) - 1.0*sin(theta5) + 1.0)*(cos(theta5)*sin(theta4) + cos(theta4)*sin(theta6) - 1.0*cos(theta5)*cos(theta6)*sin(theta4)))/25,                                                                                                                                                                                                                                                                                                                                                                                                                                                                                                                                                                                                                                                                                                                                                                                                                                                                                                                                                                                                                                                                                                                                                                                                                                                                                                                                                                                                                                                                                                                                                                                                                                                               0.16*cos(theta5)^2 - 0.16*cos(theta6)^2 - 0.32*cos(theta5)^2*cos(theta6) + 0.16*cos(theta5)^2*cos(theta6)^2 + 0.46,                                                                                                                                                                                                                                                                                                                                                                                                                                                                                                                                                                                                                                                                                                                                                                                                                                                                                                                                                                                                                                                                                                                                                                              -0.4*sin(theta5)*sin(theta6)*(0.4*cos(theta6) - 0.4),                                                                                                                                                                                                                                                                                                                                                                                                                                                                                                                                                                                                                                                                                                                                                                  -(cos(theta5)*(8.0*cos(theta6) - 13.0))/50;
                                                                                                                                                                                                                                                                                                                                                                                                                                                                                                                                                                                                                                                                                                                                                                                                                                                                                                                                                                                                                                                                                                                                                                                                                                                                                                                                                                                                                                                                                                                                                                                                                                                                                                                                                                                                                                                                                                                                                                                                                                                                                                                                                                                                                                                                                                                                                                                                                                                                                                                                                                                                                                                                                                                                                                                                                                                                                                                                                                                                                                                                                                                                                                                                                                                                                                                                                                                                                                                                                                                                      0.08*cos(theta2)*sin(theta4)*sin(theta5) + 0.36*sin(theta2)*sin(theta3)*sin(theta4) - 0.36*cos(theta2)*cos(theta3)*sin(theta4) - 0.16*cos(theta2)*cos(theta3)*cos(theta6)^2*sin(theta4) + 0.16*cos(theta6)^2*sin(theta2)*sin(theta3)*sin(theta4) + 0.32*cos(theta2)*cos(theta3)*cos(theta6)*sin(theta4) + 0.16*cos(theta2)*cos(theta3)*sin(theta4)*sin(theta5) - 0.08*cos(theta2)*cos(theta6)*sin(theta4)*sin(theta5) - 0.32*cos(theta6)*sin(theta2)*sin(theta3)*sin(theta4) + 0.16*cos(theta2)*sin(theta3)*sin(theta5)*sin(theta6) + 0.16*cos(theta3)*sin(theta2)*sin(theta5)*sin(theta6) - 0.16*sin(theta2)*sin(theta3)*sin(theta4)*sin(theta5) - 0.16*cos(theta2)*cos(theta3)*cos(theta4)*cos(theta5)*sin(theta6) - 0.16*cos(theta2)*cos(theta3)*cos(theta6)*sin(theta4)*sin(theta5) + 0.16*cos(theta4)*cos(theta5)*sin(theta2)*sin(theta3)*sin(theta6) - 0.16*cos(theta2)*cos(theta6)*sin(theta3)*sin(theta5)*sin(theta6) - 0.16*cos(theta3)*cos(theta6)*sin(theta2)*sin(theta5)*sin(theta6) + 0.16*cos(theta6)*sin(theta2)*sin(theta3)*sin(theta4)*sin(theta5) + 0.16*cos(theta2)*cos(theta3)*cos(theta4)*cos(theta5)*cos(theta6)*sin(theta6) - 0.16*cos(theta4)*cos(theta5)*cos(theta6)*sin(theta2)*sin(theta3)*sin(theta6),                                                                                                                                                                                                                                                                                                                                                                                                                                                                                                                                                                                                                                                                                                                                                                                                                                                                                                                                                                                                                                                                                                                                                                                                                                                                                                                                                                                                                                                                                                                                                                                                                                                                                                                                                                                                                                                                                                                                                                                                                                                                                                                                                                                0.1*cos(theta4) + (0.4*cos(theta6) - 0.4)*(0.4*cos(theta4)*cos(theta6) - 0.4*cos(theta4) + 0.2*cos(theta5)*sin(theta3) + 0.4*cos(theta4)*sin(theta5) + 0.4*cos(theta5)*sin(theta4)*sin(theta6) + 0.2*cos(theta3)*cos(theta4)*sin(theta5)) + 0.1*cos(theta6)*(cos(theta4)*cos(theta6) + cos(theta5)*sin(theta4)*sin(theta6)) + 0.1*sin(theta6)*(cos(theta4)*sin(theta6) - 1.0*cos(theta5)*cos(theta6)*sin(theta4)),                                                                                                                                                                                                                                                                                                                                                                                                                                                                                                                                                                                                                                                                                                                                                                                                                                                                                                                                                                                                                                                                                                                                                                                                                                                                                                                                                                                                                                                                                                                                                                                                                                                                                                                                                                                                                                                                                                                                                                                                                                                                                                                                                                                        0.36*cos(theta4) - 0.32*cos(theta4)*cos(theta6) - 0.16*cos(theta4)*sin(theta5) + 0.16*cos(theta4)*cos(theta6)^2 - 0.16*cos(theta5)*sin(theta4)*sin(theta6) + 0.16*cos(theta4)*cos(theta6)*sin(theta5) + 0.16*cos(theta5)*cos(theta6)*sin(theta4)*sin(theta6),                                                                                                                                                                                                                                                                                                                                                                                                                                                                                                                                                                                                                                                                                                                                                                                                                                                                                                                                                                                                                                                                                                                                                                                                                                                                                                                                                                                                                                                                                                                                                                                                                                                                                                                             -0.4*sin(theta5)*sin(theta6)*(0.4*cos(theta6) - 0.4),                                                                                                                                                                                                                                                                                                                                                                                                                                                                                                                                                                                                                                                                                                                                                                                                                                                                                                                                                                                                                                                                                                                                                                                      0.16*cos(theta6)^2 - 0.32*cos(theta6) + 0.36,                                                                                                                                                                                                                                                                                                                                                                                                                                                                                                                                                                                                                                                                                                                                                                                                           0;
                                                                                                                                                                                                                                                                                                                                                                                                                                                                                                                                                                                                                                                                                                                                                                                                                                                                                                                                                                                                                                                                                                                                                                                                                                                                                                                                                                                                                                                                                                                                                                                                                                                                                                                                                                                                                                                                                                                                                                                                                                                                                                                                                                                                                                                                                                                                                                                                                                                                                                                                                                                                                                                                                                                                                                                                                                                                                                                                                                                                                                                                                                                                                                                                                                                                                                                                                                                                                                                                                                                                                                                                                                                                                                                                                                                                                                                                                                                                                            0.08*cos(theta2)*cos(theta4)*cos(theta6) + 0.26*cos(theta2)*cos(theta5)*sin(theta3) + 0.26*cos(theta3)*cos(theta5)*sin(theta2) + 0.16*cos(theta2)*cos(theta3)*cos(theta4)*cos(theta6) + 0.26*cos(theta2)*cos(theta3)*cos(theta4)*sin(theta5) - 0.16*cos(theta2)*cos(theta5)*cos(theta6)*sin(theta3) - 0.16*cos(theta3)*cos(theta5)*cos(theta6)*sin(theta2) - 0.16*cos(theta4)*cos(theta6)*sin(theta2)*sin(theta3) + 0.08*cos(theta2)*cos(theta5)*sin(theta4)*sin(theta6) - 0.26*cos(theta4)*sin(theta2)*sin(theta3)*sin(theta5) - 0.16*cos(theta2)*cos(theta3)*cos(theta4)*cos(theta6)*sin(theta5) + 0.16*cos(theta2)*cos(theta3)*cos(theta5)*sin(theta4)*sin(theta6) + 0.16*cos(theta4)*cos(theta6)*sin(theta2)*sin(theta3)*sin(theta5) - 0.16*cos(theta5)*sin(theta2)*sin(theta3)*sin(theta4)*sin(theta6),                                                                                                                                                                                                                                                                                                                                                                                                                                                                                                                                                                                                                                                                                                                                                                                                                                                                                                                                                                                                                                                                                                                                                                                                                                                                                                                                                                                                                                                                                                                                                                                                                                                                                                                                                                                                                                                                                                                                                                                                                                                                                                                                                                                                                                                                                                   0.16*cos(theta6)*sin(theta4) + 0.26*sin(theta4)*sin(theta5) - 0.16*cos(theta6)*sin(theta4)*sin(theta5) + 0.08*sin(theta3)*sin(theta5)*sin(theta6) + 0.08*cos(theta3)*cos(theta6)*sin(theta4) - 0.16*cos(theta4)*cos(theta5)*sin(theta6) - 0.08*cos(theta3)*cos(theta4)*cos(theta5)*sin(theta6),                                                                                                                                                                                                                                                                                                                                                                                                                                                                                                                                                                                                                                                                                                                                                                                                                                                                                                                                                                                                                                                                                                                                                                                                                                                                                                                                                                                                                                                                                                                                                                                                                                                                                                                                                                                                                                                                                                                                                                                                                                                                                                                                                                                                                                                                                                   0.16*cos(theta6)*sin(theta4) + 0.26*sin(theta4)*sin(theta5) - 0.16*cos(theta6)*sin(theta4)*sin(theta5) - 0.16*cos(theta4)*cos(theta5)*sin(theta6),                                                                                                                                                                                                                                                                                                                                                                                                                                                                                                                                                                                                                                                                                                                                                                                                                                                                                                                                                                                                                                                                                                                                                                                                                                                                                                                                                                                                                                                                                                                                                                                                                                                                                                                                       -(cos(theta5)*(8.0*cos(theta6) - 13.0))/50,                                                                                                                                                                                                                                                                                                                                                                                                                                                                                                                                                                                                                                                                                                                                                                                                                                                                                                                                                                                                                                                                                                                                                                                                                                 0,                                                                                                                                                                                                                                                                                                                                                                                                                                                                                                                                                                                                                                                                                                                                                                                                        0.26]
 
g=[7.848*cos(theta2)*sin(theta1) - 9.81*sin(theta1)*sin(theta2)*sin(theta3) + 9.81*cos(theta2)*cos(theta3)*sin(theta1) - 3.924*cos(theta1)*cos(theta5)*sin(theta4) - 3.924*cos(theta1)*cos(theta4)*sin(theta6) + 3.924*cos(theta1)*cos(theta5)*cos(theta6)*sin(theta4) - 3.924*cos(theta2)*cos(theta3)*sin(theta1)*sin(theta5) + 3.924*sin(theta1)*sin(theta2)*sin(theta3)*sin(theta5) - 3.924*cos(theta2)*cos(theta4)*cos(theta5)*sin(theta1)*sin(theta3) - 3.924*cos(theta3)*cos(theta4)*cos(theta5)*sin(theta1)*sin(theta2) + 3.924*cos(theta2)*cos(theta3)*cos(theta6)*sin(theta1)*sin(theta5) + 3.924*cos(theta2)*sin(theta1)*sin(theta3)*sin(theta4)*sin(theta6) + 3.924*cos(theta3)*sin(theta1)*sin(theta2)*sin(theta4)*sin(theta6) - 3.924*cos(theta6)*sin(theta1)*sin(theta2)*sin(theta3)*sin(theta5) + 3.924*cos(theta2)*cos(theta4)*cos(theta5)*cos(theta6)*sin(theta1)*sin(theta3) + 3.924*cos(theta3)*cos(theta4)*cos(theta5)*cos(theta6)*sin(theta1)*sin(theta2);
                                                                                                                                                                                                                                                                                                                 1.962*cos(theta1)*(4.0*sin(theta2) + 5.0*cos(theta2)*sin(theta3) + 5.0*cos(theta3)*sin(theta2) - 2.0*cos(theta2)*sin(theta3)*sin(theta5) - 2.0*cos(theta3)*sin(theta2)*sin(theta5) + 2.0*cos(theta2)*cos(theta3)*cos(theta4)*cos(theta5) - 2.0*cos(theta4)*cos(theta5)*sin(theta2)*sin(theta3) - 2.0*cos(theta2)*cos(theta3)*sin(theta4)*sin(theta6) + 2.0*cos(theta2)*cos(theta6)*sin(theta3)*sin(theta5) + 2.0*cos(theta3)*cos(theta6)*sin(theta2)*sin(theta5) + 2.0*sin(theta2)*sin(theta3)*sin(theta4)*sin(theta6) - 2.0*cos(theta2)*cos(theta3)*cos(theta4)*cos(theta5)*cos(theta6) + 2.0*cos(theta4)*cos(theta5)*cos(theta6)*sin(theta2)*sin(theta3));
                                                                                                                                                                                                                                                                                                                                   1.962*cos(theta1)*(5.0*cos(theta2)*sin(theta3) + 5.0*cos(theta3)*sin(theta2) - 2.0*cos(theta2)*sin(theta3)*sin(theta5) - 2.0*cos(theta3)*sin(theta2)*sin(theta5) + 2.0*cos(theta2)*cos(theta3)*cos(theta4)*cos(theta5) - 2.0*cos(theta4)*cos(theta5)*sin(theta2)*sin(theta3) - 2.0*cos(theta2)*cos(theta3)*sin(theta4)*sin(theta6) + 2.0*cos(theta2)*cos(theta6)*sin(theta3)*sin(theta5) + 2.0*cos(theta3)*cos(theta6)*sin(theta2)*sin(theta5) + 2.0*sin(theta2)*sin(theta3)*sin(theta4)*sin(theta6) - 2.0*cos(theta2)*cos(theta3)*cos(theta4)*cos(theta5)*cos(theta6) + 2.0*cos(theta4)*cos(theta5)*cos(theta6)*sin(theta2)*sin(theta3));
                                                                                                                                                                                                                                                                                                                                                                               3.924*sin(theta1)*sin(theta4)*sin(theta6) - 3.924*cos(theta4)*cos(theta5)*sin(theta1) + 3.924*cos(theta4)*cos(theta5)*cos(theta6)*sin(theta1) - 3.924*cos(theta1)*cos(theta2)*cos(theta5)*sin(theta3)*sin(theta4) - 3.924*cos(theta1)*cos(theta3)*cos(theta5)*sin(theta2)*sin(theta4) - 3.924*cos(theta1)*cos(theta2)*cos(theta4)*sin(theta3)*sin(theta6) - 3.924*cos(theta1)*cos(theta3)*cos(theta4)*sin(theta2)*sin(theta6) + 3.924*cos(theta1)*cos(theta2)*cos(theta5)*cos(theta6)*sin(theta3)*sin(theta4) + 3.924*cos(theta1)*cos(theta3)*cos(theta5)*cos(theta6)*sin(theta2)*sin(theta4);
                                                                                                                                                                                                                                                                                                                                                                                                                                                                                                                                                                                                                                                                             9.81*cos(theta1)*(0.4*cos(theta6) - 0.4)*(cos(theta5)*sin(theta2)*sin(theta3) - 1.0*cos(theta2)*cos(theta3)*cos(theta5) + cos(theta2)*cos(theta4)*sin(theta3)*sin(theta5) + cos(theta3)*cos(theta4)*sin(theta2)*sin(theta5)) - 9.81*sin(theta1)*sin(theta4)*sin(theta5)*(0.4*cos(theta6) - 0.4);
                                                                                                                                                                                                                                                                                                                                                                                                                                                                                                                               3.924*cos(theta1)*(cos(theta2)*cos(theta6)*sin(theta3)*sin(theta4) + cos(theta3)*cos(theta6)*sin(theta2)*sin(theta4) - cos(theta2)*cos(theta3)*sin(theta5)*sin(theta6) + sin(theta2)*sin(theta3)*sin(theta5)*sin(theta6) - cos(theta2)*cos(theta4)*cos(theta5)*sin(theta3)*sin(theta6) - cos(theta3)*cos(theta4)*cos(theta5)*sin(theta2)*sin(theta6)) + (981*sin(theta1)*(cos(theta4)*cos(theta6) + cos(theta5)*sin(theta4)*sin(theta6)))/250];
 
                                                                                                                                                                                                                                                                                                                                                                                                                                                                                                               
